simulink model "sim2"  (R2022a)
settings: Solver=VariableStepAuto  StartTime=0.0  StopTime=10.0  RelTol=1e-3
libraries: dspstat3 x20, dspadpt3 x6
settings Model: Creator=targi  LastModifiedBy=targi

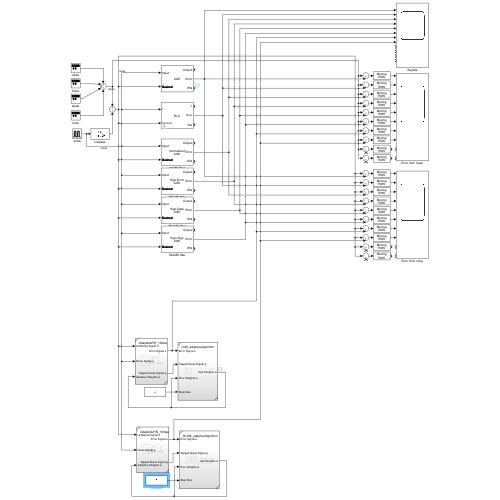
[thumbnail: Simulink's stored preview of the top-level diagram]
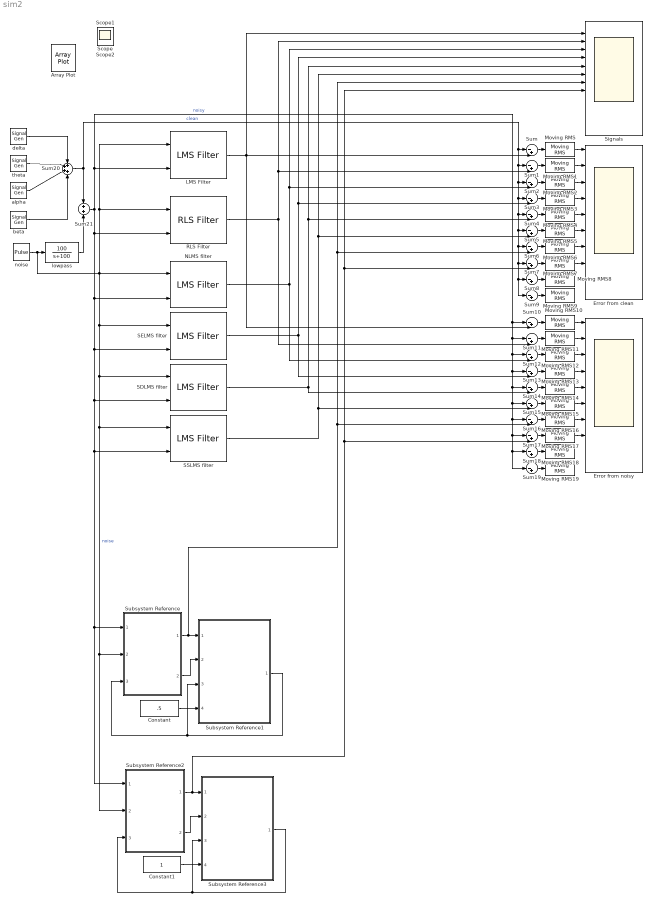
== system sim2 ==
  Constant : Constant  Value=.5
  Constant1 : Constant
  Error from clean : Scope  NumInputPorts=10
  Error from noisy : Scope  NumInputPorts=10
  LMS Filter : dspadpt3/LMS Filter  Algo=LMS  L=32  stepflag=Dialog  mu=0.1  leakage=1.0  ic=0  Adapt=off  resetflag=None  weights=on  addnparflag=off  roundingMode=Floor  overflowMode=off
      settings: SourceProductBaseCode=DS
  Moving RMS{,1..19} (20 alike) : dspstat3/Moving RMS  Method=Sliding window  ForgettingFactorPort=off  SpecifyWindowLength=on  WindowLength=50  ForgettingFactor=0.9  SimulateUsing=Code generation
      settings: SourceProductBaseCode=DS
  NLMS filter : dspadpt3/LMS Filter  Algo=Normalized LMS  L=32  stepflag=Dialog  mu=0.1  leakage=1.0  ic=0  Adapt=off  resetflag=None  weights=on  addnparflag=off  roundingMode=Floor  overflowMode=off
      settings: SourceProductBaseCode=DS
  RLS Filter : dspadpt3/RLS Filter  L=32  lambdaflag=Dialog  lambda=1.0  addnparflag=on  ic=0  delta=0.1  Adapt=off  resetflag=None  weights=on
      settings: SourceProductBaseCode=DS
  SDLMS filter : dspadpt3/LMS Filter  Algo=Sign-Data LMS  L=32  stepflag=Dialog  mu=0.1  leakage=1.0  ic=0  Adapt=off  resetflag=None  weights=on  addnparflag=off  roundingMode=Floor  overflowMode=off
      settings: SourceProductBaseCode=DS
  SELMS filter : dspadpt3/LMS Filter  Algo=Sign-Error LMS  L=32  stepflag=Dialog  mu=0.01  leakage=1.0  ic=0  Adapt=off  resetflag=None  weights=on  addnparflag=off  roundingMode=Floor  overflowMode=off
      settings: SourceProductBaseCode=DS
  SSLMS filter : dspadpt3/LMS Filter  Algo=Sign-Sign LMS  L=32  stepflag=Dialog  mu=0.01  leakage=1.0  ic=0  Adapt=off  resetflag=None  weights=on  addnparflag=off  roundingMode=Floor  overflowMode=off
      settings: SourceProductBaseCode=DS
  Signals : Scope  NumInputPorts=12
  Subsystem Reference : Subsystem  ReferencedSubsystem=AdaptibleFIR_100taps
  Subsystem Reference1 : Subsystem  ReferencedSubsystem=LMS_adaptiveAlgorithm
  Subsystem Reference2 : Subsystem  ReferencedSubsystem=AdaptibleFIR_100taps
  Subsystem Reference3 : Subsystem  ReferencedSubsystem=DLMS_adaptiveAlgorithm
  Sum{,1..19} (20 alike) : Sum  Inputs=|-+
  Sum20 : Sum  Inputs=++++
  Sum21 : Sum  Inputs=+|+
  alpha : SignalGenerator  Amplitude=.002  Frequency=10
  beta : SignalGenerator  Amplitude=.001  Frequency=22
  delta : SignalGenerator  Amplitude=.004  Frequency=2
  lowpass : TransferFcn  Numerator=[100]  Denominator=[1 100]
  noise : DiscretePulseGenerator  PulseType=Time based  Period=.4  PulseWidth=5
  theta : SignalGenerator  Amplitude=.003  Frequency=6
  Array Plot : ArrayPlot  IOType=viewer  WindowPosition=[636.000000,337.000000,800.000000,500.000000,]  IsFloating=on  ScopeFrameLocation=window  DefaultConfigurationName=dsp.scopes.ArrayPlotBlockSpecification
  Scope : Scope
  Scope1 : Scope
  Scope2 : Scope
  wires:
  Moving RMS/1 -> Error from clean/1
  Moving RMS1/1 -> Error from clean/2
  Sum/1 -> Moving RMS/1
  Sum1/1 -> Moving RMS1/1
  Sum2/1 -> Moving RMS2/1
  Sum3/1 -> Moving RMS3/1
  Sum4/1 -> Moving RMS4/1
  Sum5/1 -> Moving RMS5/1
  Sum6/1 -> Moving RMS6/1
  Sum7/1 -> Moving RMS7/1
  Sum8/1 -> Moving RMS8/1
  Sum9/1 -> Moving RMS9/1
  Sum19/1 -> Moving RMS19/1
  Sum18/1 -> Moving RMS18/1
  Sum17/1 -> Moving RMS17/1
  Sum16/1 -> Moving RMS16/1
  Sum15/1 -> Moving RMS15/1
  Sum14/1 -> Moving RMS14/1
  Sum13/1 -> Moving RMS13/1
  Sum12/1 -> Moving RMS12/1
  Sum11/1 -> Moving RMS11/1
  Sum10/1 -> Moving RMS10/1
  delta/1 -> Sum20/1
  noise/1 -> RLS Filter/1, LMS Filter/1, Subsystem Reference2/2, Subsystem Reference/2, SSLMS filter/1, SDLMS filter/1, SELMS filter/1, NLMS filter/1, lowpass/1  "noise"
  lowpass/1 -> Sum21/2
  theta/1 -> Sum20/2
  Sum20/1 -> Sum21/1, Sum9/1, Sum8/1, Sum7/1, Sum6/1, Sum5/1, Sum4/1, Sum3/1, Sum2/1, Sum1/1, Sum/1  "clean"
  beta/1 -> Sum20/4
  alpha/1 -> Sum20/3
  Sum21/1 -> Sum19/1, Sum18/1, Sum17/1, Sum16/1, Sum15/1, Sum14/1, Sum13/1, Sum12/1, Sum11/1, Sum10/1, LMS Filter/2, Subsystem Reference2/1, Subsystem Reference/1, SSLMS filter/2, SDLMS filter/2, SELMS filter/2, NLMS filter/2, RLS Filter/2  "noisy"
  LMS Filter/2 -> Sum10/2, Signals/1, Sum/2
  RLS Filter/2 -> Sum11/2, Signals/2, Sum1/2
  Moving RMS10/1 -> Error from noisy/1
  Moving RMS11/1 -> Error from noisy/2
  Subsystem Reference/1 -> Subsystem Reference1/1, Sum16/2, Sum6/2, Signals/7
  Subsystem Reference/2 -> Subsystem Reference1/2
  Subsystem Reference1/1 -> Subsystem Reference1/3, Subsystem Reference/3
  Constant/1 -> Subsystem Reference1/4
  NLMS filter/2 -> Sum12/2, Sum2/2, Signals/3
  SELMS filter/2 -> Sum13/2, Sum3/2, Signals/4
  SDLMS filter/2 -> Sum14/2, Sum4/2, Signals/5
  SSLMS filter/2 -> Sum15/2, Sum5/2, Signals/6
  Moving RMS2/1 -> Error from clean/3
  Moving RMS3/1 -> Error from clean/4
  Moving RMS4/1 -> Error from clean/5
  Moving RMS5/1 -> Error from clean/6
  Moving RMS12/1 -> Error from noisy/3
  Moving RMS13/1 -> Error from noisy/4
  Moving RMS14/1 -> Error from noisy/5
  Moving RMS15/1 -> Error from noisy/6
  Moving RMS6/1 -> Error from clean/7
  Moving RMS16/1 -> Error from noisy/7
  Constant1/1 -> Subsystem Reference3/4
  Subsystem Reference2/2 -> Subsystem Reference3/2
  Subsystem Reference2/1 -> Sum17/2, Sum7/2, Signals/8, Subsystem Reference3/1
  Subsystem Reference3/1 -> Subsystem Reference3/3, Subsystem Reference2/3
  Moving RMS7/1 -> Error from clean/8
  Moving RMS17/1 -> Error from noisy/8
